simulink model "IIR_DFormI"  (R2023a)
settings: Solver=VariableStepDiscrete  StartTime=0.0  StopTime=20000  RelTol=1e-3
PreLoadFcn:
  | IIR_DFormI_PreLoadFcn
undefined symbols (not defined in the file): a1, a2, b0, b1, b2, data_binary_pt, data_width, Fs
libraries: hdlBasic x38, dspstat3 x2, hdlUtilities x1, dspswit3 x1, simulink x1, dspsrcs4 x1, vmcUtilities x1
settings Model: Creator=alexc  LastModifiedBy=robg
settings SolverCC: AlgebraicLoopSolver=TrustRegion
settings DataIOCC: LimitDataPoints=on  SaveFormat=Array  SignalLoggingSaveFormat=ModelDataLogs  ReturnWorkspaceOutputs=off  SignalLoggingName=sigsOut
settings OptimizationCC: BlockReduction=off  BooleanDataType=off  DefaultParameterBehavior=Inlined  ExpressionDepthLimit=2147483647  InitFltsAndDblsToZero=on  LifeSpan=inf
settings DebuggingCC: SaveWithParameterizedLinksMsg=none  UnderspecifiedInitializationDetection=Classic  MergeDetectMultiDrivingBlocksExec=none  SignalResolutionControl=TryResolveAllWithWarning  MultiTaskDSMMsg=warning  MultiTaskCondExecSysMsg=none  FcnCallInpInsideContextMsg=warning  UnconnectedInputMsg=warning  UnconnectedOutputMsg=warning  UnconnectedLineMsg=warning  AllowSymbolicDim=off  StateNameClashWarn=warning  SFUnexpectedBacktrackingDiag=warning  SFNoUnconditionalDefaultTransitionDiag=warning  SFExecutionAtInitializationDiag=none  ArithmeticOperatorsInVariantConditions=warning
settings HardwareCC: ProdBitPerPointer=32  ProdBitPerSizeT=32  ProdBitPerPtrDiffT=32  ProdLargestAtomicFloat=None  ProdIntDivRoundTo=Undefined  ProdEndianess=Unspecified  ProdWordSize=32  ProdHWDeviceType=32-bit Generic  TargetUnknown=on
settings ModelReferenceCC: EnableRefExpFcnMdlSchedulingChecks=on  PropagateSignalLabelsOutOfModel=off
settings SFSimCC: SimUseLocalCustomCode=off  CustomCodeUndefinedFunction=UseInterfaceOnly
settings RTWCC: RTWUseLocalCustomCode=off  DLArmComputeVersion=19.05
settings CodeAppCC: StateflowObjectComments=on
settings GRTTargetCC: TargetFcnLib=ansi_tfl_tmw.mat  TargetLangStandard=C89/C90 (ANSI)  CombineOutputUpdateFcns=off  GRTInterface=on
settings ConfigComp: CovMetricSettings=dw  CovSaveCumulativeToWorkspaceVar=on  CovSaveSingleToWorkspaceVar=on  CovExternalEMLEnable=off

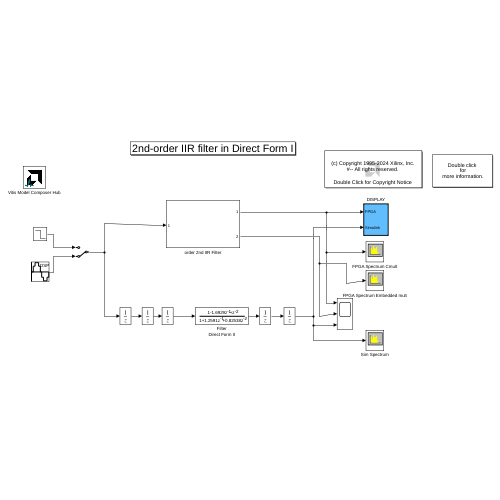
[thumbnail: Simulink's stored preview of the top-level diagram]
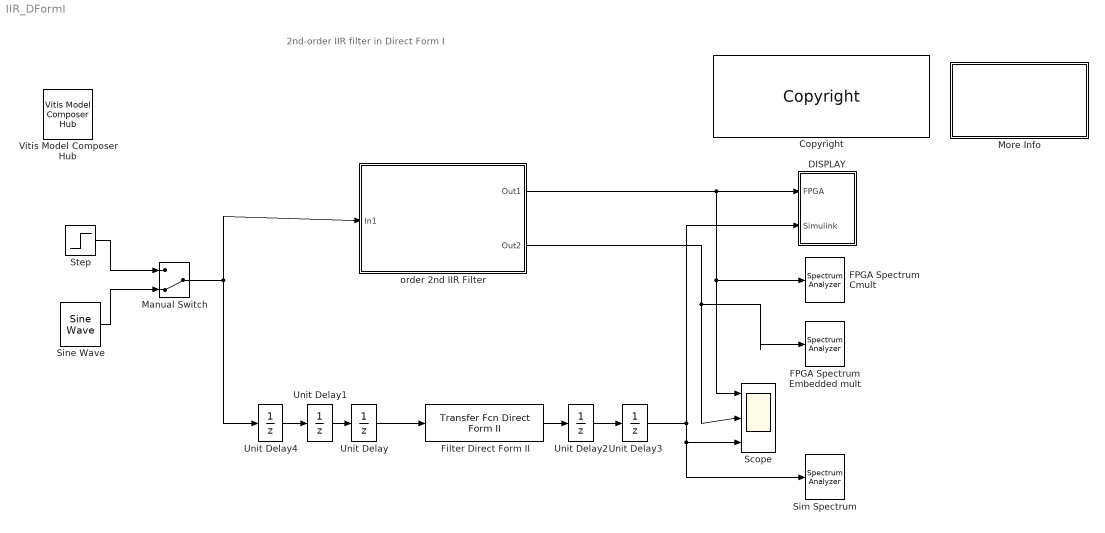
== system IIR_DFormI ==
  note: 2nd-order IIR filter in Direct Form I
  Copyright : hdlUtilities/Copyright  copyrighttext="Copyright (c) 2024  by  Xilinx, Inc. All rights reserved.<br><br>This file contains proprietary, confidential information of Xilinx, Inc., is distributed under license from Xilinx, Inc., and may be used, copied and/or disclosed only pursuant to the terms of a valid license agreement with Xilinx, Inc. Xilinx hereby grants you a license to use this file solely for design, simulation, implementation and creation of design files limited to Xilinx devices or technologies. Use with non-Xilinx devices or technologies is expressly prohibited and immediately terminates your license unless covered by a separate agreement.<br><br>Xilinx is providing this design, code, or information \"as-is\" solely for use in developing programs and solutions for Xilinx devices, with no obligation on the part of Xilinx to provide support. By providing this design, code, or information as one possible implementation of this feature, application or standard, Xilinx is making no representation that this implementation is free from any claims of infringement. You are responsible for obtaining any rights you may require for your implementation. Xilinx expressly disclaims any warranty whatsoever with respect to the adequacy of the implementation, including but not limited to any warranties or representations that this implementation is free from claims of infringement, implied warranties of merchantability or fitness for a particular purpose.<br><br>Xilinx products are not intended for use in life support appliances, devices, or systems. Use in such applications is expressly prohibited.<br><br>Any modifications that are made to the Source Code are done at the user's sole risk and will be unsupported.<br><br>This copyright and support notice must be retained as part of this text at all times. (c) Copyright 1995-2024 Xilinx, Inc. All rights reserved."  block_type=copyright
  DISPLAY : Subsystem  TreatAsAtomicUnit=on
  FPGA Spectrum Cmult : SpectrumAnalyzer  WindowPosition=[465 290 423 236]  Visible=on  SpectrumType=Power density  Method=Welch  SampleRate=1  PlotAsTwoSidedSpectrum=off  RBWSource=Property  RBW=0.00293262012  FFTLength=128  Span=0.5  CenterFrequency=0.25  StartFrequency=0  StopFrequency=0.5  AveragingMethod=Exponential  YLabel=Magnitude  YLimits=[-419.8492,73.7242]  ChannelNames="[\"\"]"  DefaultConfigurationName=spbscopes.SpectrumAnalyzerBlockCfg
  FPGA Spectrum Embedded mult : SpectrumAnalyzer  WindowPosition=[1002 398 423 236]  Visible=on  SpectrumType=Power density  Method=Welch  SampleRate=1  PlotAsTwoSidedSpectrum=off  RBWSource=Property  RBW=0.00293262012  FFTLength=128  Span=0.5  CenterFrequency=0.25  StartFrequency=0  StopFrequency=0.5  AveragingMethod=Exponential  YLabel=Magnitude  YLimits=[-3637.3349,405.3922]  ChannelNames="[\"\"]"  DefaultConfigurationName=spbscopes.SpectrumAnalyzerBlockCfg
  Filter Direct Form II : simulink/Additional Math & Discrete/Additional Discrete/Transfer Fcn Direct Form II  NumCoefVec=[1 -1.6929 1]  DenCoefVec=[1.2591 0.82538]  vinit=0.0  DoSatur=off
  Manual Switch : ManualSwitch  CurrentSetting=0
  More Info : Subsystem
      mask Display: disp('Double click\n for\n more information.')
  Scope : Scope  NumInputPorts=3
  Sim Spectrum : SpectrumAnalyzer  WindowPosition=[458 283 437 227]  Visible=on  SpectrumType=Power density  Method=Welch  SampleRate=1  PlotAsTwoSidedSpectrum=off  RBWSource=Property  RBW=0.00293262012  FFTLength=128  Span=0.5  CenterFrequency=0.25  StartFrequency=0  StopFrequency=0.5  AveragingMethod=Exponential  YLabel=Magnitude  YLimits=[-374.0793,42.8241]  ChannelNames="[\"\"]"  DefaultConfigurationName=spbscopes.SpectrumAnalyzerBlockCfg
  Sine Wave : dspsrcs4/Sine Wave  Amplitude=0.99  Frequency=1/32  Phase=0  SampleMode=Discrete  OutComplex=Real  CompMethod=Trigonometric fcn  TableSize=Speed  SampleTime=1/Fs  SamplesPerFrame=1  ResetState=Restart at time zero  OutputFrames=on  dataType=double  wordLen=16  udDataType=sfix(16)  fracBitsMode=Best precision  numFracBits=14  OutDataTypeStr=double  LastOutDataTypeStr=double
  Step : Step  Before=1  After=0  SampleTime=1
  Unit Delay{,1..4} (5 alike) : UnitDelay  SampleTime=Fs  HasFrameUpgradeWarning=on
  Vitis Model Composer Hub : vmcUtilities/Vitis Model Composer Hub  Tag=genX  CodeGeneration=off  StartColumn=1  NumberOfColumns=1  TargetDirectory=./code  exportDesign=off  analyzeDesign=off  validateDesignOnHw=off  ExportType=System Generator  IpVendor=xilinx.com  IpLibrary=hls  IpVersion=1.0  IpHWLanguage=Verilog  AieCompilerOptions={}  AieSimulatorOptions={}  CreateTestbench=off  TestbenchStackSize=10  RunRtlSim=off  RunCSim=off  RunAieSim=off  AieSimTimeout=50000  RunAieSimProfiling=off  LaunchVitisAnalyzer=off  PlotOutput=off  RunX86Sim=off  X86SimTimeout=10  GenHwImage=off  GenLibadfXo=off  GenHwValidationCode=off  PlatformType=Not Specified  HwSystemType=Baremetal  HwValidationTarget=hw  ProjDevice=xcku11p-ffva1156-1-e  ProjDevicePart=xcku11p-ffva1156-1-e  SamplePeriod=-1  ClockFrequency=200  DataPathParallelism=1  xilinxfamily=kintexuplus  part=xcku11p  speed=-1-e  package=ffva1156  directory=./netlist  testbench=off  incr_netlist=off  synthesis_tool=Vivado  clock_wrapper=Clock Enables  dbl_ovrd=According to Block Masks  dcm_input_clock_period=10  sysclk_period=16  simulink_period=Fs  eval_field=0  LogFileName=''  NThreads=4
  order 2nd IIR Filter : Subsystem
  wires:
  Unit Delay/1 -> Filter Direct Form II/1
  Filter Direct Form II/1 -> Unit Delay2/1
  Sine Wave/1 -> Manual Switch/2
  Step/1 -> Manual Switch/1
  Manual Switch/1 -> order 2nd IIR Filter/1(In1), Unit Delay4/1
  Unit Delay1/1 -> Unit Delay/1
  Unit Delay2/1 -> Unit Delay3/1
  Unit Delay3/1 -> DISPLAY/2(Simulink), Sim Spectrum/1, Scope/3
  Unit Delay4/1 -> Unit Delay1/1
  order 2nd IIR Filter/1(Out1) -> FPGA Spectrum Cmult/1, Scope/1, DISPLAY/1(FPGA)
  order 2nd IIR Filter/2(Out2) -> Scope/2, FPGA Spectrum Embedded mult/1

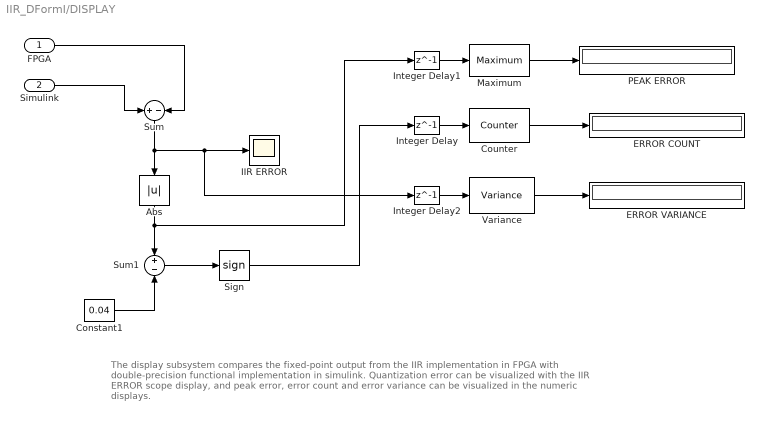
== system IIR_DFormI/DISPLAY ==
  note: The display subsystem compares the fixed-point output from the IIR implementation in FPGA
      | with double-precision functional implementation in simulink. Quantization error can be visualized
      | with the IIR ERROR scope display, and peak error, error count and error variance can be visualized
      | in the numeric displays.
  FPGA : Inport
  Simulink : Inport  Port=2
  Abs : Abs
  Constant1 : Constant  Value=0.04
  Counter : dspswit3/Counter  Direction=Up  CountEvent=Rising edge  CounterSize=User defined  MaxCount=200000000  InitialCount=0  Output=Count  HitValue=32  ResetInput=off  SamplesPerFrame=1  Ts=1  CntDtype=double  HitDtype=Logical
  ERROR COUNT : Display
      settings: Format=long_e
  ERROR VARIANCE : Display
      settings: Format=long_e
  IIR ERROR : Scope
  Integer Delay : Delay  DelayLength=1  InitialCondition=0  UseCircularBuffer=on
  Integer Delay1 : Delay  DelayLength=1  InitialCondition=0  UseCircularBuffer=on
  Integer Delay2 : Delay  DelayLength=1  InitialCondition=0  UseCircularBuffer=on
  Maximum : dspstat3/Maximum  operation=maximum  fcn=Running  indexBase=One  operateOver=Each column  Dimension=1  reset=None  roiEnable=off  roiType=Rectangles  roiPortion=Entire ROI  roiOutput=Individual statistics for each ROI  roiFlag=off  roundingMode=Floor  overflowMode=off  accumDataTypeStr=Inherit: Same as product output  accumLastDataTypeStr=Inherit: Same as product output
  PEAK ERROR : Display
      settings: Format=long_e
  Sign : Signum
  Sum : Sum  Inputs=+-  InputSameDT=on  SaturateOnIntegerOverflow=on  OutDataTypeStr=Inherit: Same as first input
  Sum1 : Sum  Inputs=+-  InputSameDT=on  SaturateOnIntegerOverflow=on  OutDataTypeStr=Inherit: Same as first input
  Variance : dspstat3/Variance  run=on  reset_popup=None  directionMode=Each column  dimension=1  roiEnable=off  roiType=Rectangles  roiPortion=Entire ROI  roiOutput=Individual statistics for each ROI  roiFlag=off  roundingMode=Floor  overflowMode=off
  wires:
  FPGA/1 -> Sum/2
  Simulink/1 -> Sum/1
  Sum/1 -> Abs/1, IIR ERROR/1, Integer Delay2/1
  Constant1/1 -> Sum1/2
  Abs/1 -> Sum1/1, Integer Delay1/1
  Sum1/1 -> Sign/1
  Sign/1 -> Integer Delay/1
  Counter/1 -> ERROR COUNT/1
  Variance/1 -> ERROR VARIANCE/1
  Maximum/1 -> PEAK ERROR/1
  Integer Delay/1 -> Counter/1
  Integer Delay1/1 -> Maximum/1
  Integer Delay2/1 -> Variance/1

== system IIR_DFormI/More Info ==
  note: This design example shows two distinct FPGA implementations of a 2nd order IIR filter in Direct Form I,
      | and compares them to the double precision Simulink IIR filter block.
      |
      | IIR_Cmult is implemented using constant coefficient multipliers implemented in LUTs
      |
      | IIR_mult is implemented using embedded multipliers. This approach can only be used
      | with the FPGAs that provide the embedded multipliers.
      |
      | Multiple display blocks allow the user to visualize the Power Spectrum  Density (PSD) of each
      | implementation as well as the quantization error in the DISPLAY block.
      |
      | All the variables such as data width, coefficient width, Sample period, and coefficient values are
      | initialized in the sysgenIIR_PreLoadFcn.m file. The default setting use 12 bit data and coefficients
  note: 2nd-order IIR filter in Direct Form I

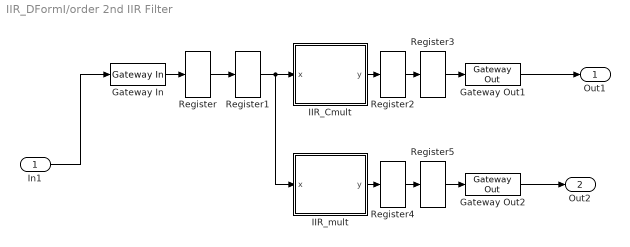
== system IIR_DFormI/order 2nd IIR Filter ==
  In1 : Inport
  Gateway In : hdlBasic/Gateway In  gui_display_data_type=Fixed-point  arith_type=Signed (2's comp)  n_bits=data_width  bin_pt=data_binary_pt  preci_type=Single  exp_width=8  frac_width=24  rows=1  columns=1  quantization="Round  (unbiased: +/- Inf)"  overflow=Saturate  period=Fs  UseAsADC=off  ADCChannel='1'  interface=None  automatic_assignment=on  address_offset=hex2dec('00')  intf_name=''  intf_description=''  default_value=0  timing_constraint=None  locs_specified=off  LOCs={}  io_standard={}  inherit_from_input=off  hdl_port=on  XmcBlockStatus=1  maskContainerNames=group4  block_type=gatewayin  block_config=sysgen:gateway_in_config  block_width_w=590  block_height_w=620  block_width=640  block_height=850
  Gateway Out1 : hdlBasic/Gateway Out  inherit_from_input=off  hdl_port=on  rows=1  columns=1  UseAsDAC=off  DACChannel='1'  interface=None  automatic_assignment=on  address_offset=hex2dec('00')  intf_name=''  intf_description=''  timing_constraint=None  locs_specified=off  LOCs={}  io_standard={}  XmcBlockStatus=1  maskContainerNames=group4  block_type=gatewayout  block_config=sysgen:gateway_out_config  block_width_w=590  block_height_w=620  block_width=620  block_height=750
  Gateway Out2 : hdlBasic/Gateway Out  inherit_from_input=off  hdl_port=on  rows=1  columns=1  UseAsDAC=off  DACChannel='1'  interface=None  automatic_assignment=on  address_offset=hex2dec('00')  intf_name=''  intf_description=''  timing_constraint=None  locs_specified=off  LOCs={}  io_standard={}  XmcBlockStatus=1  maskContainerNames=group4  block_type=gatewayout  block_config=sysgen:gateway_out_config  block_width_w=590  block_height_w=620  block_width=620  block_height=750
  IIR_Cmult : Subsystem
  IIR_mult : Subsystem
  Register{,1..5} (6 alike) : hdlBasic/Register  init=0  rst=off  en=off  XmcBlockStatus=1  maskContainerNames=tabcontainer1  block_type=register  block_config=sysgen:Register_config
  Out1 : Outport
  Out2 : Outport  Port=2
  wires:
  Register/1 -> Register1/1
  Gateway Out2/1 -> Out2/1
  Register3/1 -> Gateway Out1/1
  IIR_Cmult/1(y) -> Register2/1
  IIR_mult/1(y) -> Register4/1
  In1/1 -> Gateway In/1
  Register1/1 -> IIR_Cmult/1(x), IIR_mult/1(x)
  Gateway In/1 -> Register/1
  Register5/1 -> Gateway Out2/1
  Register2/1 -> Register3/1
  Gateway Out1/1 -> Out1/1
  Register4/1 -> Register5/1

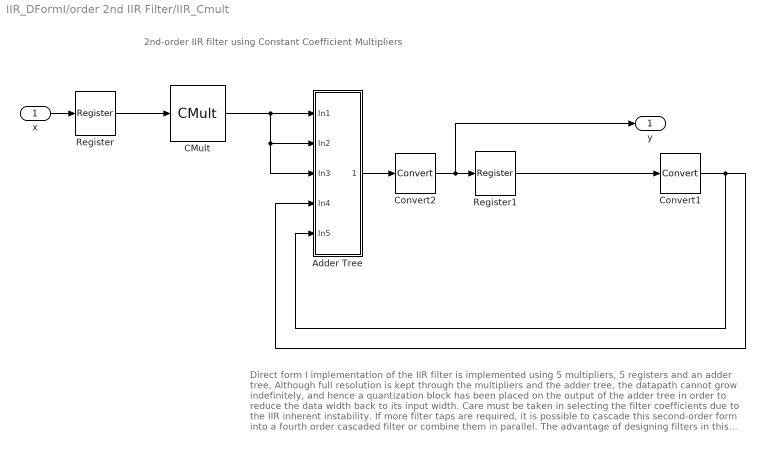
== system IIR_DFormI/order 2nd IIR Filter/IIR_Cmult ==
  note: Direct form I implementation of the IIR filter is implemented using 5 multipliers, 5 registers
      | and an adder tree, Although full resolution is kept through the multipliers and the
      | adder tree, the datapath cannot grow indefinitely, and hence a quantization block has
      | been placed on the output of the adder tree in order to reduce the data width back to its
      | input width.
      | Care must be taken in selecting the filter coefficients due to the IIR inherent instability.
      |
      | If more filter taps are required, it is possible to cascade this second-order form into a
      | fourth order cascaded filter or combine them in parallel. The advantage of designing
      | filters in this way is that they are modular, which makes their implementation much simpler.
      |
      | In IIR_Cmult, we chose to use constant coefficient multipliers which are very efficiently
      | implemented in LUTs. Partial products are currently saved in distributed memories,
      | but an option in the CMult block allows the user to target Block Memories if necessary.
      | Because of the feedback loop, no latency and hence no pipelining is possible in this design. It is for this reason, fairly
      | difficult to achieve high sample rate with such implementation. On the other hand, it is
      | possible to reduce the size and performance by processing the data sequentially instead of
      | in parallel as currently shown in this example.
  note: 2nd-order IIR filter using Constant Coefficient Multipliers
  x : Inport
  Adder Tree : Subsystem
  CMult : hdlBasic/CMult  const=b0  gui_display_data_type=Fixed-point  const_n_bits=coef_width  const_bin_pt=coef_binary_pt  float_type=Single  exp_bits=8  fraction_bits=24  en=off  latency=0  precision=Full  arith_type="Signed  (2's comp)"  n_bits=8  bin_pt=6  quantization="Round  (unbiased: +/- Inf)"  overflow=Wrap  use_behavioral_HDL=off  mem_type=Distributed RAM  pipeline=off  use_rpm=off  placement_style=Rectangular Shape  XmcBlockStatus=1  maskContainerNames=tabcontainer1  block_type=cmult  block_config=sysgen:CMult_config
      settings: infoedit=[]
  Convert1 : hdlBasic/Convert  gui_display_data_type=Fixed-point  arith_type=Signed (2's comp)  n_bits=data_width+12  bin_pt=data_binary_pt+10  float_type=Single  exp_bits=8  fraction_bits=24  quantization=Truncate  overflow=Saturate  en=off  latency=0  pipeline=off  XmcBlockStatus=1  maskContainerNames=group2  block_type=convert  block_config=sysgen:Convert_config  block_width=595  block_height=885
  Convert2 : hdlBasic/Convert  gui_display_data_type=Fixed-point  arith_type=Signed (2's comp)  n_bits=data_width  bin_pt=data_binary_pt  float_type=Single  exp_bits=8  fraction_bits=24  quantization=Truncate  overflow=Saturate  en=off  latency=0  pipeline=off  XmcBlockStatus=1  maskContainerNames=group2  block_type=convert  block_config=sysgen:Convert_config  block_width=595  block_height=885
  Register : hdlBasic/Register  init=0  rst=off  en=off  XmcBlockStatus=1  maskContainerNames=tabcontainer1  block_type=register  block_config=sysgen:Register_config
  Register1 : hdlBasic/Register  init=0  rst=off  en=off  XmcBlockStatus=1  maskContainerNames=tabcontainer1  block_type=register  block_config=sysgen:Register_config
  y : Outport  VectorParamsAs1DForOutWhenUnconnected=off
  wires:
  Register/1 -> CMult/1
  CMult/1 -> Adder Tree/1(In1), Adder Tree/2(In2), Adder Tree/3(In3)
  Adder Tree/1(Out1) -> Convert2/1
  Register1/1 -> Convert1/1
  x/1 -> Register/1
  Convert2/1 -> Register1/1, y/1
  Convert1/1 -> Adder Tree/4(In4), Adder Tree/5(In5)

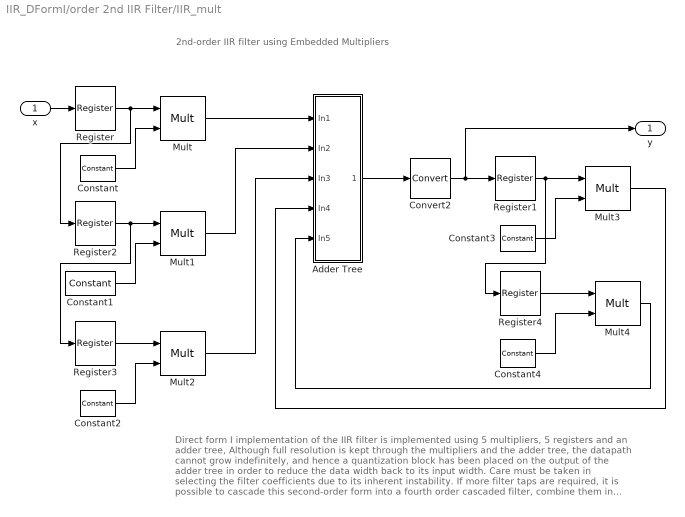
== system IIR_DFormI/order 2nd IIR Filter/IIR_mult ==
  note: Direct form I implementation of the IIR filter is implemented using 5 multipliers, 5 registers
      | and an adder tree, Although full resolution is kept through the multipliers and the
      | adder tree, the datapath cannot grow indefinitely, and hence a quantization block has
      | been placed on the output of the adder tree in order to reduce the data width back to its
      | input width.
      | Care must be taken in selecting the filter coefficients due to its inherent instability.
      |
      | If more filter taps are required, it is possible to cascade this second-order form into a
      | fourth order cascaded filter, combine them in parallel or time share the current design
      | by saving multiple sets of coefficients in distributed memories. Similarly, the time sharing
      | approach can be used for multi-channel requirements, in which case, the coefficients can
      | be saved in distributed memories or block memories depending on the number of channels.
      |
      | Because of the feedback loop, no latency and hence no pipelining is possible in this design.
      | It is for this reason, fairly difficult to achieve high sample rate with such implementation.
  note: 2nd-order IIR filter using Embedded Multipliers
  x : Inport
  Adder Tree : Subsystem
  Constant : hdlBasic/Constant  const=b0  gui_display_data_type=Fixed-point  arith_type=Signed (2's comp)  n_bits=coef_width  bin_pt=coef_binary_pt  preci_type=Single  exp_width=8  frac_width=24  explicit_period=off  period=1  XmcBlockStatus=1  maskContainerNames=tabcontainer1  block_type=constant  block_config=sysgen:Constant_config
  Constant1 : hdlBasic/Constant  const=b1  gui_display_data_type=Fixed-point  arith_type=Signed (2's comp)  n_bits=coef_width  bin_pt=coef_binary_pt  preci_type=Single  exp_width=8  frac_width=24  explicit_period=off  period=1  XmcBlockStatus=1  maskContainerNames=tabcontainer1  block_type=constant  block_config=sysgen:Constant_config
  Constant2 : hdlBasic/Constant  const=b2  gui_display_data_type=Fixed-point  arith_type=Signed (2's comp)  n_bits=coef_width  bin_pt=coef_binary_pt  preci_type=Single  exp_width=8  frac_width=24  explicit_period=off  period=1  XmcBlockStatus=1  maskContainerNames=tabcontainer1  block_type=constant  block_config=sysgen:Constant_config
  Constant3 : hdlBasic/Constant  const=-a1  gui_display_data_type=Fixed-point  arith_type=Signed (2's comp)  n_bits=coef_width  bin_pt=coef_binary_pt  preci_type=Single  exp_width=8  frac_width=24  explicit_period=off  period=1  XmcBlockStatus=1  maskContainerNames=tabcontainer1  block_type=constant  block_config=sysgen:Constant_config
  Constant4 : hdlBasic/Constant  const=-a2  gui_display_data_type=Fixed-point  arith_type=Signed (2's comp)  n_bits=coef_width  bin_pt=coef_binary_pt  preci_type=Single  exp_width=8  frac_width=24  explicit_period=off  period=1  XmcBlockStatus=1  maskContainerNames=tabcontainer1  block_type=constant  block_config=sysgen:Constant_config
  Convert2 : hdlBasic/Convert  gui_display_data_type=Fixed-point  arith_type=Signed (2's comp)  n_bits=data_width  bin_pt=data_binary_pt  float_type=Single  exp_bits=8  fraction_bits=24  quantization=Truncate  overflow=Saturate  en=off  latency=0  pipeline=off  XmcBlockStatus=1  maskContainerNames=group2  block_type=convert  block_config=sysgen:Convert_config  block_width=595  block_height=885
  Mult{,1..4} (5 alike) : hdlBasic/Mult  precision=Full  arith_type="Signed  (2's comp)"  n_bits=8  bin_pt=2  quantization=Truncate  overflow=Wrap  en=off  latency=0  opt_float=off  fp_mult_usage=No Usage  use_behavioral_HDL=off  opt=Speed  use_embedded=on  optimum_pipeline=off  pipeline=off  use_rpm=off  placement_style=Rectangular shape  XmcBlockStatus=1  maskContainerNames=group1  block_type=mult  block_config=sysgen:Mult_config  block_width=598  block_height=876
  Register{,1..4} (5 alike) : hdlBasic/Register  init=0  rst=off  en=off  XmcBlockStatus=1  maskContainerNames=tabcontainer1  block_type=register  block_config=sysgen:Register_config
  y : Outport  VectorParamsAs1DForOutWhenUnconnected=off
  wires:
  x/1 -> Register/1
  Register1/1 -> Mult3/1, Register4/1
  Constant3/1 -> Mult3/2
  Convert2/1 -> y/1, Register1/1
  Mult4/1 -> Adder Tree/5(In5)
  Mult3/1 -> Adder Tree/4(In4)
  Constant4/1 -> Mult4/2
  Register4/1 -> Mult4/1
  Mult2/1 -> Adder Tree/3(In3)
  Constant2/1 -> Mult2/2
  Register3/1 -> Mult2/1
  Constant1/1 -> Mult1/2
  Register2/1 -> Register3/1, Mult1/1
  Constant/1 -> Mult/2
  Register/1 -> Register2/1, Mult/1
  Mult1/1 -> Adder Tree/2(In2)
  Mult/1 -> Adder Tree/1(In1)
  Adder Tree/1(Out1) -> Convert2/1

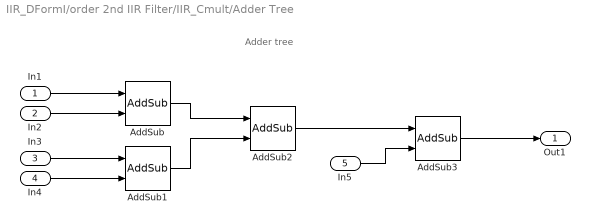
== system IIR_DFormI/order 2nd IIR Filter/IIR_Cmult/Adder Tree ==
  note: Adder tree
  In1 : Inport
  In2 : Inport  Port=2
  In3 : Inport  Port=3
  In4 : Inport  Port=4
  In5 : Inport  Port=5
  AddSub : hdlBasic/AddSub  mode=Addition  use_carryin=off  use_carryout=off  en=off  latency=0  precision=Full  arith_type=Unsigned  n_bits=8  bin_pt=2  quantization=Truncate  overflow=Wrap  use_behavioral_HDL=off  hw_selection=Fabric  pipelined=off  use_rpm=off  XmcBlockStatus=1  maskContainerNames=tabcontainer1  block_type=addsub  block_config=sysgen:Addsub_config
  AddSub1 : hdlBasic/AddSub  mode=Addition  use_carryin=off  use_carryout=off  en=off  latency=0  precision=Full  arith_type=Unsigned  n_bits=8  bin_pt=2  quantization=Truncate  overflow=Wrap  use_behavioral_HDL=on  hw_selection=Fabric  pipelined=off  use_rpm=off  XmcBlockStatus=1  maskContainerNames=tabcontainer1  block_type=addsub  block_config=sysgen:Addsub_config
  AddSub2 : hdlBasic/AddSub  mode=Addition  use_carryin=off  use_carryout=off  en=off  latency=0  precision=Full  arith_type=Unsigned  n_bits=8  bin_pt=2  quantization=Truncate  overflow=Wrap  use_behavioral_HDL=on  hw_selection=Fabric  pipelined=off  use_rpm=off  XmcBlockStatus=1  maskContainerNames=tabcontainer1  block_type=addsub  block_config=sysgen:Addsub_config
  AddSub3 : hdlBasic/AddSub  mode=Addition  use_carryin=off  use_carryout=off  en=off  latency=0  precision=Full  arith_type=Unsigned  n_bits=8  bin_pt=2  quantization=Truncate  overflow=Wrap  use_behavioral_HDL=off  hw_selection=Fabric  pipelined=off  use_rpm=off  XmcBlockStatus=1  maskContainerNames=tabcontainer1  block_type=addsub  block_config=sysgen:Addsub_config
  Out1 : Outport  VectorParamsAs1DForOutWhenUnconnected=off
  wires:
  In1/1 -> AddSub/1
  In2/1 -> AddSub/2
  In5/1 -> AddSub3/2
  AddSub3/1 -> Out1/1
  In3/1 -> AddSub1/1
  In4/1 -> AddSub1/2
  AddSub/1 -> AddSub2/1
  AddSub1/1 -> AddSub2/2
  AddSub2/1 -> AddSub3/1

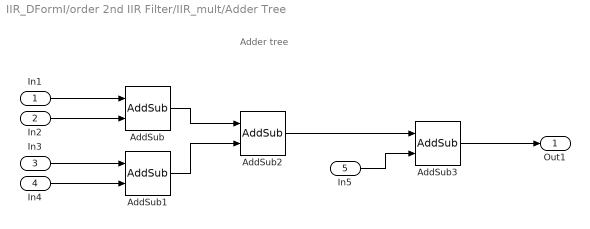
== system IIR_DFormI/order 2nd IIR Filter/IIR_mult/Adder Tree ==
  note: Adder tree
  In1 : Inport
  In2 : Inport  Port=2
  In3 : Inport  Port=3
  In4 : Inport  Port=4
  In5 : Inport  Port=5
  AddSub : hdlBasic/AddSub  mode=Addition  use_carryin=off  use_carryout=off  en=off  latency=0  precision=Full  arith_type=Unsigned  n_bits=8  bin_pt=2  quantization=Truncate  overflow=Wrap  use_behavioral_HDL=off  hw_selection=Fabric  pipelined=off  use_rpm=off  XmcBlockStatus=1  maskContainerNames=tabcontainer1  block_type=addsub  block_config=sysgen:Addsub_config
  AddSub1 : hdlBasic/AddSub  mode=Addition  use_carryin=off  use_carryout=off  en=off  latency=0  precision=Full  arith_type=Unsigned  n_bits=8  bin_pt=2  quantization=Truncate  overflow=Wrap  use_behavioral_HDL=on  hw_selection=Fabric  pipelined=off  use_rpm=off  XmcBlockStatus=1  maskContainerNames=tabcontainer1  block_type=addsub  block_config=sysgen:Addsub_config
  AddSub2 : hdlBasic/AddSub  mode=Addition  use_carryin=off  use_carryout=off  en=off  latency=0  precision=Full  arith_type=Unsigned  n_bits=8  bin_pt=2  quantization=Truncate  overflow=Wrap  use_behavioral_HDL=on  hw_selection=Fabric  pipelined=off  use_rpm=off  XmcBlockStatus=1  maskContainerNames=tabcontainer1  block_type=addsub  block_config=sysgen:Addsub_config
  AddSub3 : hdlBasic/AddSub  mode=Addition  use_carryin=off  use_carryout=off  en=off  latency=0  precision=Full  arith_type=Unsigned  n_bits=8  bin_pt=2  quantization=Truncate  overflow=Wrap  use_behavioral_HDL=off  hw_selection=Fabric  pipelined=off  use_rpm=off  XmcBlockStatus=1  maskContainerNames=tabcontainer1  block_type=addsub  block_config=sysgen:Addsub_config
  Out1 : Outport  VectorParamsAs1DForOutWhenUnconnected=off
  wires:
  In1/1 -> AddSub/1
  In2/1 -> AddSub/2
  In5/1 -> AddSub3/2
  AddSub3/1 -> Out1/1
  In3/1 -> AddSub1/1
  In4/1 -> AddSub1/2
  AddSub/1 -> AddSub2/1
  AddSub1/1 -> AddSub2/2
  AddSub2/1 -> AddSub3/1
